simulink model "AN_Simulink_Model_v1_fil"  (R2019b)
settings: Solver=VariableStepAuto  StartTime=0.0  StopTime=testtime  RelTol=1e-3
InitFcn:
  | AN_InitFcn_Callback
StopFcn:
  | AN_StopFcn_Callback
undefined symbols (not defined in the file or in its folder): tdres
libraries: hdlmdlgenlib x193, simulink x4, fillib x1, dspsrcs4 x1
(part 4 of 6)

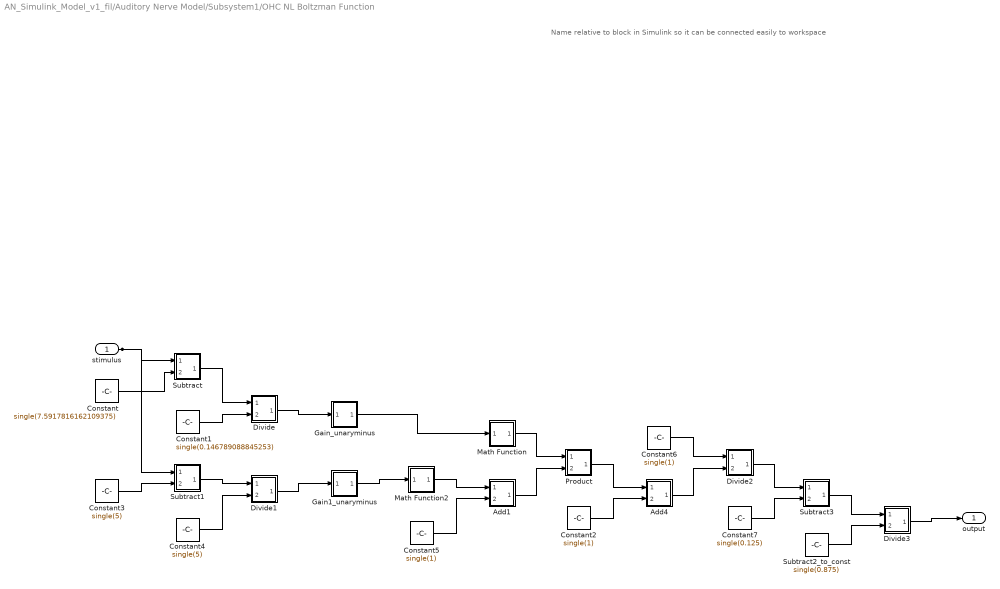
== system AN_Simulink_Model_v1_fil/Auditory Nerve Model/Subsystem1/OHC NL Boltzman Function ==
  note: Name relative to block in Simulink so it can be connected easily to workspace
  stimulus : Inport  OutDataTypeStr=single  PortDimensions=1  SampleTime=2.08333333333333e-05
  Add1 : Subsystem
      mask Display: disp('NFP\nadd');
  Add4 : Subsystem
      mask Display: disp('NFP\nadd');
  Constant : Constant  Value=single(7.5917816162109375)  OutDataTypeStr=single  SampleTime=-1
  Constant1 : Constant  Value=single(0.146789088845253)  OutDataTypeStr=single  SampleTime=-1
  Constant2 : Constant  Value=single(1)  OutDataTypeStr=single  SampleTime=-1
  Constant3 : Constant  Value=single(5)  OutDataTypeStr=single  SampleTime=-1
  Constant4 : Constant  Value=single(5)  OutDataTypeStr=single  SampleTime=-1
  Constant5 : Constant  Value=single(1)  OutDataTypeStr=single  SampleTime=-1
  Constant6 : Constant  Value=single(1)  OutDataTypeStr=single  SampleTime=-1
  Constant7 : Constant  Value=single(0.125)  OutDataTypeStr=single  SampleTime=-1
  Divide : Subsystem
      mask Display: disp('NFP\nmul');
  Divide1 : Subsystem
      mask Display: disp('NFP\nmul');
  Divide2 : Subsystem
      mask Display: disp('NFP\nmul');
  Divide3 : Subsystem
      mask Display: disp('NFP\nmul');
  Gain1_unaryminus : Subsystem
      mask Display: disp('NFP\numinus');
  Gain_unaryminus : Subsystem
      mask Display: disp('NFP\numinus');
  Math Function : Subsystem
      mask Display: disp('NFP\nmath');
  Math Function2 : Subsystem
      mask Display: disp('NFP\nmath');
  Product : Subsystem
      mask Display: disp('NFP\nmul');
  Subtract : Subsystem
      mask Display: disp('NFP\nadd');
  Subtract1 : Subsystem
      mask Display: disp('NFP\nadd');
  Subtract2_to_const : Constant  Value=single(0.875)  OutDataTypeStr=single  SampleTime=-1
  Subtract3 : Subsystem
      mask Display: disp('NFP\nadd');
  output : Outport  VectorParamsAs1DForOutWhenUnconnected=off
  wires:
  Subtract3/1(Out1) -> Divide3/1(In1)
  Subtract1/1(Out1) -> Divide1/1(In1)
  Subtract/1(Out1) -> Divide/1(In1)
  Product/1(Out1) -> Add4/1(In1)
  Math Function2/1(Out1) -> Add1/1(In1)
  Math Function/1(Out1) -> Product/1(In1)
  Divide3/1(Out1) -> output/1
  Divide2/1(Out1) -> Subtract3/1(In1)
  Divide1/1(Out1) -> Gain1_unaryminus/1(In1)
  Divide/1(Out1) -> Gain_unaryminus/1(In1)
  Add4/1(Out1) -> Divide2/2(In2)
  Add1/1(Out1) -> Product/2(In2)
  Gain1_unaryminus/1(Out1) -> Math Function2/1(In1)
  Gain_unaryminus/1(Out1) -> Math Function/1(In1)
  Subtract2_to_const/1 -> Divide3/2(In2)
  Constant7/1 -> Subtract3/2(In2)
  Constant6/1 -> Divide2/1(In1)
  Constant5/1 -> Add1/2(In2)
  Constant4/1 -> Divide1/2(In2)
  Constant3/1 -> Subtract1/2(In2)
  Constant2/1 -> Add4/2(In2)
  Constant1/1 -> Divide/2(In2)
  Constant/1 -> Subtract/2(In2)
  stimulus/1 -> Subtract/1(In1), Subtract1/1(In1)

== system AN_Simulink_Model_v1_fil/Compare/Assert_ihcout/RelErrCheck ==
  In1 : Inport
  In2 : Inport  Port=2
  "RelativeErrorCheck " : MATLAB Function  TreatAsAtomicUnit=on
  Out1 : Outport  VectorParamsAs1DForOutWhenUnconnected=off
  wires:
  In2/1 -> "RelativeErrorCheck "/2(R)
  In1/1 -> "RelativeErrorCheck "/1(P)
  "RelativeErrorCheck "/1(y) -> Out1/1

== system AN_Simulink_Model_v1_fil/Auditory Nerve Model/C1 Chirp Filter/C1 FIlter/Gain10_unaryminus ==
  In1 : Inport
  Gain10_unaryminus : UnaryMinus  SampleTime=2.08333333333333e-05
  Out1 : Outport
  wires:
  Gain10_unaryminus/1 -> Out1/1
  In1/1 -> Gain10_unaryminus/1

== system AN_Simulink_Model_v1_fil/Auditory Nerve Model/C1 Chirp Filter/C1 FIlter/Gain11_unaryminus ==
  In1 : Inport
  Gain11_unaryminus : UnaryMinus  SampleTime=2.08333333333333e-05
  Out1 : Outport
  wires:
  Gain11_unaryminus/1 -> Out1/1
  In1/1 -> Gain11_unaryminus/1

== system AN_Simulink_Model_v1_fil/Auditory Nerve Model/C1 Chirp Filter/C1 FIlter/Gain1_unaryminus ==
  In1 : Inport
  Gain1_unaryminus : UnaryMinus  SampleTime=2.08333333333333e-05
  Out1 : Outport
  wires:
  Gain1_unaryminus/1 -> Out1/1
  In1/1 -> Gain1_unaryminus/1

== system AN_Simulink_Model_v1_fil/Auditory Nerve Model/C1 Chirp Filter/C1 FIlter/Gain2_unaryminus ==
  In1 : Inport
  Gain2_unaryminus : UnaryMinus  SampleTime=2.08333333333333e-05
  Out1 : Outport
  wires:
  Gain2_unaryminus/1 -> Out1/1
  In1/1 -> Gain2_unaryminus/1

== system AN_Simulink_Model_v1_fil/Auditory Nerve Model/C1 Chirp Filter/C1 FIlter/Gain3_unaryminus ==
  In1 : Inport
  Gain3_unaryminus : UnaryMinus  SampleTime=2.08333333333333e-05
  Out1 : Outport
  wires:
  Gain3_unaryminus/1 -> Out1/1
  In1/1 -> Gain3_unaryminus/1

== system AN_Simulink_Model_v1_fil/Auditory Nerve Model/C1 Chirp Filter/C1 FIlter/Gain4_unaryminus ==
  In1 : Inport
  Gain4_unaryminus : UnaryMinus  SampleTime=2.08333333333333e-05
  Out1 : Outport
  wires:
  Gain4_unaryminus/1 -> Out1/1
  In1/1 -> Gain4_unaryminus/1

== system AN_Simulink_Model_v1_fil/Auditory Nerve Model/C1 Chirp Filter/C1 FIlter/Gain5_unaryminus ==
  In1 : Inport
  Gain5_unaryminus : UnaryMinus  SampleTime=2.08333333333333e-05
  Out1 : Outport
  wires:
  Gain5_unaryminus/1 -> Out1/1
  In1/1 -> Gain5_unaryminus/1

== system AN_Simulink_Model_v1_fil/Auditory Nerve Model/C1 Chirp Filter/C1 FIlter/Gain7_unaryminus ==
  In1 : Inport
  Gain7_unaryminus : UnaryMinus  SampleTime=2.08333333333333e-05
  Out1 : Outport
  wires:
  Gain7_unaryminus/1 -> Out1/1
  In1/1 -> Gain7_unaryminus/1

== system AN_Simulink_Model_v1_fil/Auditory Nerve Model/C1 Chirp Filter/C1 FIlter/Gain8_unaryminus ==
  In1 : Inport
  Gain8_unaryminus : UnaryMinus  SampleTime=2.08333333333333e-05
  Out1 : Outport
  wires:
  Gain8_unaryminus/1 -> Out1/1
  In1/1 -> Gain8_unaryminus/1

== system AN_Simulink_Model_v1_fil/Auditory Nerve Model/C1 Chirp Filter/C1 FIlter/Gain9_unaryminus ==
  In1 : Inport
  Gain9_unaryminus : UnaryMinus  SampleTime=2.08333333333333e-05
  Out1 : Outport
  wires:
  Gain9_unaryminus/1 -> Out1/1
  In1/1 -> Gain9_unaryminus/1

== system AN_Simulink_Model_v1_fil/Auditory Nerve Model/C1 Chirp Filter/C1 FIlter/Product ==
  In1 : Inport
  In2 : Inport  Port=2
  Product : Product  Inputs=**  OutDataTypeStr=single  SampleTime=2.08333333333333e-05
  Out1 : Outport
  wires:
  Product/1 -> Out1/1
  In2/1 -> Product/2
  In1/1 -> Product/1

== system AN_Simulink_Model_v1_fil/Auditory Nerve Model/C1 Chirp Filter/C1 FIlter/Product1 ==
  In1 : Inport
  In2 : Inport  Port=2
  Product1 : Product  Inputs=**  OutDataTypeStr=single  SampleTime=2.08333333333333e-05
  Out1 : Outport
  wires:
  Product1/1 -> Out1/1
  In2/1 -> Product1/2
  In1/1 -> Product1/1

== system AN_Simulink_Model_v1_fil/Auditory Nerve Model/C1 Chirp Filter/C1 FIlter/Product10 ==
  In1 : Inport
  In2 : Inport  Port=2
  Product10 : Product  Inputs=**  OutDataTypeStr=single  SampleTime=2.08333333333333e-05
  Out1 : Outport
  wires:
  Product10/1 -> Out1/1
  In2/1 -> Product10/2
  In1/1 -> Product10/1

== system AN_Simulink_Model_v1_fil/Auditory Nerve Model/C1 Chirp Filter/C1 FIlter/Product11 ==
  In1 : Inport
  In2 : Inport  Port=2
  Product11 : Product  Inputs=**  OutDataTypeStr=single  SampleTime=2.08333333333333e-05
  Out1 : Outport
  wires:
  Product11/1 -> Out1/1
  In2/1 -> Product11/2
  In1/1 -> Product11/1

== system AN_Simulink_Model_v1_fil/Auditory Nerve Model/C1 Chirp Filter/C1 FIlter/Product12 ==
  In1 : Inport
  In2 : Inport  Port=2
  Product12 : Product  Inputs=**  OutDataTypeStr=single  SampleTime=2.08333333333333e-05
  Out1 : Outport
  wires:
  Product12/1 -> Out1/1
  In2/1 -> Product12/2
  In1/1 -> Product12/1

== system AN_Simulink_Model_v1_fil/Auditory Nerve Model/C1 Chirp Filter/C1 FIlter/Product13 ==
  In1 : Inport
  In2 : Inport  Port=2
  Product13 : Product  Inputs=**  OutDataTypeStr=single  SampleTime=2.08333333333333e-05
  Out1 : Outport
  wires:
  Product13/1 -> Out1/1
  In2/1 -> Product13/2
  In1/1 -> Product13/1

== system AN_Simulink_Model_v1_fil/Auditory Nerve Model/C1 Chirp Filter/C1 FIlter/Product14 ==
  In1 : Inport
  In2 : Inport  Port=2
  Product14 : Product  Inputs=**  OutDataTypeStr=single  SampleTime=2.08333333333333e-05
  Out1 : Outport
  wires:
  Product14/1 -> Out1/1
  In2/1 -> Product14/2
  In1/1 -> Product14/1

== system AN_Simulink_Model_v1_fil/Auditory Nerve Model/C1 Chirp Filter/C1 FIlter/Product15 ==
  In1 : Inport
  In2 : Inport  Port=2
  Product15 : Product  Inputs=**  OutDataTypeStr=single  SampleTime=2.08333333333333e-05
  Out1 : Outport
  wires:
  Product15/1 -> Out1/1
  In2/1 -> Product15/2
  In1/1 -> Product15/1

== system AN_Simulink_Model_v1_fil/Auditory Nerve Model/C1 Chirp Filter/C1 FIlter/Product16 ==
  In1 : Inport
  In2 : Inport  Port=2
  Product16 : Product  Inputs=**  OutDataTypeStr=single  SampleTime=2.08333333333333e-05
  Out1 : Outport
  wires:
  Product16/1 -> Out1/1
  In2/1 -> Product16/2
  In1/1 -> Product16/1

== system AN_Simulink_Model_v1_fil/Auditory Nerve Model/C1 Chirp Filter/C1 FIlter/Product17 ==
  In1 : Inport
  In2 : Inport  Port=2
  Product17 : Product  Inputs=**  OutDataTypeStr=single  SampleTime=2.08333333333333e-05
  Out1 : Outport
  wires:
  Product17/1 -> Out1/1
  In2/1 -> Product17/2
  In1/1 -> Product17/1

== system AN_Simulink_Model_v1_fil/Auditory Nerve Model/C1 Chirp Filter/C1 FIlter/Product18 ==
  In1 : Inport
  In2 : Inport  Port=2
  Product18 : Product  Inputs=**  OutDataTypeStr=single  SampleTime=2.08333333333333e-05
  Out1 : Outport
  wires:
  Product18/1 -> Out1/1
  In2/1 -> Product18/2
  In1/1 -> Product18/1

== system AN_Simulink_Model_v1_fil/Auditory Nerve Model/C1 Chirp Filter/C1 FIlter/Product19 ==
  In1 : Inport
  In2 : Inport  Port=2
  Product19 : Product  Inputs=**  OutDataTypeStr=single  SampleTime=2.08333333333333e-05
  Out1 : Outport
  wires:
  Product19/1 -> Out1/1
  In2/1 -> Product19/2
  In1/1 -> Product19/1

== system AN_Simulink_Model_v1_fil/Auditory Nerve Model/C1 Chirp Filter/C1 FIlter/Product2 ==
  In1 : Inport
  In2 : Inport  Port=2
  Product2 : Product  Inputs=**  OutDataTypeStr=single  SampleTime=2.08333333333333e-05
  Out1 : Outport
  wires:
  Product2/1 -> Out1/1
  In2/1 -> Product2/2
  In1/1 -> Product2/1

== system AN_Simulink_Model_v1_fil/Auditory Nerve Model/C1 Chirp Filter/C1 FIlter/Product20 ==
  In1 : Inport
  In2 : Inport  Port=2
  Product20 : Product  Inputs=**  OutDataTypeStr=single  SampleTime=2.08333333333333e-05
  Out1 : Outport
  wires:
  Product20/1 -> Out1/1
  In2/1 -> Product20/2
  In1/1 -> Product20/1

== system AN_Simulink_Model_v1_fil/Auditory Nerve Model/C1 Chirp Filter/C1 FIlter/Product21 ==
  In1 : Inport
  In2 : Inport  Port=2
  Product21 : Product  Inputs=**  OutDataTypeStr=single  SampleTime=2.08333333333333e-05
  Out1 : Outport
  wires:
  Product21/1 -> Out1/1
  In2/1 -> Product21/2
  In1/1 -> Product21/1

== system AN_Simulink_Model_v1_fil/Auditory Nerve Model/C1 Chirp Filter/C1 FIlter/Product22 ==
  In1 : Inport
  In2 : Inport  Port=2
  Product22 : Product  Inputs=**  OutDataTypeStr=single  SampleTime=2.08333333333333e-05
  Out1 : Outport
  wires:
  Product22/1 -> Out1/1
  In2/1 -> Product22/2
  In1/1 -> Product22/1

== system AN_Simulink_Model_v1_fil/Auditory Nerve Model/C1 Chirp Filter/C1 FIlter/Product23 ==
  In1 : Inport
  In2 : Inport  Port=2
  Product23 : Product  Inputs=**  OutDataTypeStr=single  SampleTime=2.08333333333333e-05
  Out1 : Outport
  wires:
  Product23/1 -> Out1/1
  In2/1 -> Product23/2
  In1/1 -> Product23/1

== system AN_Simulink_Model_v1_fil/Auditory Nerve Model/C1 Chirp Filter/C1 FIlter/Product24 ==
  In1 : Inport
  In2 : Inport  Port=2
  Product24 : Product  Inputs=**  OutDataTypeStr=single  SampleTime=2.08333333333333e-05
  Out1 : Outport
  wires:
  Product24/1 -> Out1/1
  In2/1 -> Product24/2
  In1/1 -> Product24/1

== system AN_Simulink_Model_v1_fil/Auditory Nerve Model/C1 Chirp Filter/C1 FIlter/Product25_to_gain ==
  In1 : Inport
  Product25_to_gain : Gain  Gain=single(0.25)
  Out1 : Outport
  wires:
  Product25_to_gain/1 -> Out1/1
  In1/1 -> Product25_to_gain/1

== system AN_Simulink_Model_v1_fil/Auditory Nerve Model/C1 Chirp Filter/C1 FIlter/Product26 ==
  In1 : Inport
  In2 : Inport  Port=2
  Product26 : Product  Inputs=**  OutDataTypeStr=single  SampleTime=2.08333333333333e-05
  Out1 : Outport
  wires:
  Product26/1 -> Out1/1
  In2/1 -> Product26/2
  In1/1 -> Product26/1

== system AN_Simulink_Model_v1_fil/Auditory Nerve Model/C1 Chirp Filter/C1 FIlter/Product3 ==
  In1 : Inport
  In2 : Inport  Port=2
  Product3 : Product  Inputs=**  OutDataTypeStr=single  SampleTime=2.08333333333333e-05
  Out1 : Outport
  wires:
  Product3/1 -> Out1/1
  In2/1 -> Product3/2
  In1/1 -> Product3/1

== system AN_Simulink_Model_v1_fil/Auditory Nerve Model/C1 Chirp Filter/C1 FIlter/Product4 ==
  In1 : Inport
  In2 : Inport  Port=2
  Product4 : Product  Inputs=**  OutDataTypeStr=single  SampleTime=2.08333333333333e-05
  Out1 : Outport
  wires:
  Product4/1 -> Out1/1
  In2/1 -> Product4/2
  In1/1 -> Product4/1

== system AN_Simulink_Model_v1_fil/Auditory Nerve Model/C1 Chirp Filter/C1 FIlter/Product5 ==
  In1 : Inport
  In2 : Inport  Port=2
  Product5 : Product  Inputs=**  OutDataTypeStr=single  SampleTime=2.08333333333333e-05
  Out1 : Outport
  wires:
  Product5/1 -> Out1/1
  In2/1 -> Product5/2
  In1/1 -> Product5/1

== system AN_Simulink_Model_v1_fil/Auditory Nerve Model/C1 Chirp Filter/C1 FIlter/Product6 ==
  In1 : Inport
  In2 : Inport  Port=2
  Product6 : Product  Inputs=**  OutDataTypeStr=single  SampleTime=2.08333333333333e-05
  Out1 : Outport
  wires:
  Product6/1 -> Out1/1
  In2/1 -> Product6/2
  In1/1 -> Product6/1

== system AN_Simulink_Model_v1_fil/Auditory Nerve Model/C1 Chirp Filter/C1 FIlter/Product7 ==
  In1 : Inport
  In2 : Inport  Port=2
  Product7 : Product  Inputs=**  OutDataTypeStr=single  SampleTime=2.08333333333333e-05
  Out1 : Outport
  wires:
  Product7/1 -> Out1/1
  In2/1 -> Product7/2
  In1/1 -> Product7/1

== system AN_Simulink_Model_v1_fil/Auditory Nerve Model/C1 Chirp Filter/C1 FIlter/Product8 ==
  In1 : Inport
  In2 : Inport  Port=2
  Product8 : Product  Inputs=**  OutDataTypeStr=single  SampleTime=2.08333333333333e-05
  Out1 : Outport
  wires:
  Product8/1 -> Out1/1
  In2/1 -> Product8/2
  In1/1 -> Product8/1

== system AN_Simulink_Model_v1_fil/Auditory Nerve Model/C1 Chirp Filter/C1 FIlter/Product9 ==
  In1 : Inport
  In2 : Inport  Port=2
  Product9 : Product  Inputs=**  OutDataTypeStr=single  SampleTime=2.08333333333333e-05
  Out1 : Outport
  wires:
  Product9/1 -> Out1/1
  In2/1 -> Product9/2
  In1/1 -> Product9/1

== system AN_Simulink_Model_v1_fil/Auditory Nerve Model/C1 Chirp Filter/C1 FIlter/Sum ==
  In1 : Inport
  In2 : Inport  Port=2
  Sum : Sum  OutDataTypeStr=single  SampleTime=2.08333333333333e-05  SaturateOnIntegerOverflow=on  InputSameDT=on
  Out1 : Outport
  wires:
  Sum/1 -> Out1/1
  In2/1 -> Sum/2
  In1/1 -> Sum/1

== system AN_Simulink_Model_v1_fil/Auditory Nerve Model/C1 Chirp Filter/C1 FIlter/Sum1 ==
  In1 : Inport
  In2 : Inport  Port=2
  Sum1 : Sum  OutDataTypeStr=single  SampleTime=2.08333333333333e-05  SaturateOnIntegerOverflow=on  InputSameDT=on
  Out1 : Outport
  wires:
  Sum1/1 -> Out1/1
  In2/1 -> Sum1/2
  In1/1 -> Sum1/1

== system AN_Simulink_Model_v1_fil/Auditory Nerve Model/C1 Chirp Filter/C1 FIlter/Sum10 ==
  In1 : Inport
  In2 : Inport  Port=2
  Sum10 : Sum  OutDataTypeStr=single  SampleTime=2.08333333333333e-05  SaturateOnIntegerOverflow=on  InputSameDT=on
  Out1 : Outport
  wires:
  Sum10/1 -> Out1/1
  In2/1 -> Sum10/2
  In1/1 -> Sum10/1

== system AN_Simulink_Model_v1_fil/Auditory Nerve Model/C1 Chirp Filter/C1 FIlter/Sum11 ==
  In1 : Inport
  In2 : Inport  Port=2
  Sum11 : Sum  OutDataTypeStr=single  SampleTime=2.08333333333333e-05  SaturateOnIntegerOverflow=on  InputSameDT=on
  Out1 : Outport
  wires:
  Sum11/1 -> Out1/1
  In2/1 -> Sum11/2
  In1/1 -> Sum11/1

== system AN_Simulink_Model_v1_fil/Auditory Nerve Model/C1 Chirp Filter/C1 FIlter/Sum12 ==
  In1 : Inport
  In2 : Inport  Port=2
  Sum12 : Sum  OutDataTypeStr=single  SampleTime=2.08333333333333e-05  SaturateOnIntegerOverflow=on  InputSameDT=on
  Out1 : Outport
  wires:
  Sum12/1 -> Out1/1
  In2/1 -> Sum12/2
  In1/1 -> Sum12/1

== system AN_Simulink_Model_v1_fil/Auditory Nerve Model/C1 Chirp Filter/C1 FIlter/Sum13 ==
  In1 : Inport
  In2 : Inport  Port=2
  Sum13 : Sum  OutDataTypeStr=single  SampleTime=2.08333333333333e-05  SaturateOnIntegerOverflow=on  InputSameDT=on
  Out1 : Outport
  wires:
  Sum13/1 -> Out1/1
  In2/1 -> Sum13/2
  In1/1 -> Sum13/1

== system AN_Simulink_Model_v1_fil/Auditory Nerve Model/C1 Chirp Filter/C1 FIlter/Sum14 ==
  In1 : Inport
  In2 : Inport  Port=2
  Sum14 : Sum  OutDataTypeStr=single  SampleTime=2.08333333333333e-05  SaturateOnIntegerOverflow=on  InputSameDT=on
  Out1 : Outport
  wires:
  Sum14/1 -> Out1/1
  In2/1 -> Sum14/2
  In1/1 -> Sum14/1

== system AN_Simulink_Model_v1_fil/Auditory Nerve Model/C1 Chirp Filter/C1 FIlter/Sum15 ==
  In1 : Inport
  In2 : Inport  Port=2
  Sum15 : Sum  OutDataTypeStr=single  SampleTime=2.08333333333333e-05  SaturateOnIntegerOverflow=on  InputSameDT=on
  Out1 : Outport
  wires:
  Sum15/1 -> Out1/1
  In2/1 -> Sum15/2
  In1/1 -> Sum15/1

== system AN_Simulink_Model_v1_fil/Auditory Nerve Model/C1 Chirp Filter/C1 FIlter/Sum16 ==
  In1 : Inport
  In2 : Inport  Port=2
  Sum16 : Sum  OutDataTypeStr=single  SampleTime=2.08333333333333e-05  SaturateOnIntegerOverflow=on  InputSameDT=on
  Out1 : Outport
  wires:
  Sum16/1 -> Out1/1
  In2/1 -> Sum16/2
  In1/1 -> Sum16/1

== system AN_Simulink_Model_v1_fil/Auditory Nerve Model/C1 Chirp Filter/C1 FIlter/Sum17 ==
  In1 : Inport
  In2 : Inport  Port=2
  Sum17 : Sum  OutDataTypeStr=single  SampleTime=2.08333333333333e-05  SaturateOnIntegerOverflow=on  InputSameDT=on
  Out1 : Outport
  wires:
  Sum17/1 -> Out1/1
  In2/1 -> Sum17/2
  In1/1 -> Sum17/1

== system AN_Simulink_Model_v1_fil/Auditory Nerve Model/C1 Chirp Filter/C1 FIlter/Sum18 ==
  In1 : Inport
  In2 : Inport  Port=2
  Sum18 : Sum  OutDataTypeStr=single  SampleTime=2.08333333333333e-05  SaturateOnIntegerOverflow=on  InputSameDT=on
  Out1 : Outport
  wires:
  Sum18/1 -> Out1/1
  In2/1 -> Sum18/2
  In1/1 -> Sum18/1

== system AN_Simulink_Model_v1_fil/Auditory Nerve Model/C1 Chirp Filter/C1 FIlter/Sum19 ==
  In1 : Inport
  In2 : Inport  Port=2
  Sum19 : Sum  OutDataTypeStr=single  SampleTime=2.08333333333333e-05  SaturateOnIntegerOverflow=on  InputSameDT=on
  Out1 : Outport
  wires:
  Sum19/1 -> Out1/1
  In2/1 -> Sum19/2
  In1/1 -> Sum19/1

== system AN_Simulink_Model_v1_fil/Auditory Nerve Model/C1 Chirp Filter/C1 FIlter/Sum2 ==
  In1 : Inport
  In2 : Inport  Port=2
  Sum2 : Sum  OutDataTypeStr=single  SampleTime=2.08333333333333e-05  SaturateOnIntegerOverflow=on  InputSameDT=on
  Out1 : Outport
  wires:
  Sum2/1 -> Out1/1
  In2/1 -> Sum2/2
  In1/1 -> Sum2/1

== system AN_Simulink_Model_v1_fil/Auditory Nerve Model/C1 Chirp Filter/C1 FIlter/Sum3 ==
  In1 : Inport
  In2 : Inport  Port=2
  Sum3 : Sum  OutDataTypeStr=single  SampleTime=2.08333333333333e-05  SaturateOnIntegerOverflow=on  InputSameDT=on
  Out1 : Outport
  wires:
  Sum3/1 -> Out1/1
  In2/1 -> Sum3/2
  In1/1 -> Sum3/1

== system AN_Simulink_Model_v1_fil/Auditory Nerve Model/C1 Chirp Filter/C1 FIlter/Sum4 ==
  In1 : Inport
  In2 : Inport  Port=2
  Sum4 : Sum  OutDataTypeStr=single  SampleTime=2.08333333333333e-05  SaturateOnIntegerOverflow=on  InputSameDT=on
  Out1 : Outport
  wires:
  Sum4/1 -> Out1/1
  In2/1 -> Sum4/2
  In1/1 -> Sum4/1

== system AN_Simulink_Model_v1_fil/Auditory Nerve Model/C1 Chirp Filter/C1 FIlter/Sum5 ==
  In1 : Inport
  In2 : Inport  Port=2
  Sum5 : Sum  OutDataTypeStr=single  SampleTime=2.08333333333333e-05  SaturateOnIntegerOverflow=on  InputSameDT=on
  Out1 : Outport
  wires:
  Sum5/1 -> Out1/1
  In2/1 -> Sum5/2
  In1/1 -> Sum5/1

== system AN_Simulink_Model_v1_fil/Auditory Nerve Model/C1 Chirp Filter/C1 FIlter/Sum6 ==
  In1 : Inport
  In2 : Inport  Port=2
  Sum6 : Sum  OutDataTypeStr=single  SampleTime=2.08333333333333e-05  SaturateOnIntegerOverflow=on  InputSameDT=on
  Out1 : Outport
  wires:
  Sum6/1 -> Out1/1
  In2/1 -> Sum6/2
  In1/1 -> Sum6/1

== system AN_Simulink_Model_v1_fil/Auditory Nerve Model/C1 Chirp Filter/C1 FIlter/Sum7 ==
  In1 : Inport
  In2 : Inport  Port=2
  Sum7 : Sum  OutDataTypeStr=single  SampleTime=2.08333333333333e-05  SaturateOnIntegerOverflow=on  InputSameDT=on
  Out1 : Outport
  wires:
  Sum7/1 -> Out1/1
  In2/1 -> Sum7/2
  In1/1 -> Sum7/1

== system AN_Simulink_Model_v1_fil/Auditory Nerve Model/C1 Chirp Filter/C1 FIlter/Sum8 ==
  In1 : Inport
  In2 : Inport  Port=2
  Sum8 : Sum  OutDataTypeStr=single  SampleTime=2.08333333333333e-05  SaturateOnIntegerOverflow=on  InputSameDT=on
  Out1 : Outport
  wires:
  Sum8/1 -> Out1/1
  In2/1 -> Sum8/2
  In1/1 -> Sum8/1

== system AN_Simulink_Model_v1_fil/Auditory Nerve Model/C1 Chirp Filter/C1 FIlter/Sum9 ==
  In1 : Inport
  In2 : Inport  Port=2
  Sum9 : Sum  OutDataTypeStr=single  SampleTime=2.08333333333333e-05  SaturateOnIntegerOverflow=on  InputSameDT=on
  Out1 : Outport
  wires:
  Sum9/1 -> Out1/1
  In2/1 -> Sum9/2
  In1/1 -> Sum9/1

== system AN_Simulink_Model_v1_fil/Auditory Nerve Model/C1 Chirp Filter/Calculate rsigma/Reciprocal1_recip ==
  In1 : Inport
  Reciprocal1_recip : Math  Operator=reciprocal  SampleTime=2.08333333333333e-05  SaturateOnIntegerOverflow=on
  Out1 : Outport
  wires:
  Reciprocal1_recip/1 -> Out1/1
  In1/1 -> Reciprocal1_recip/1

== system AN_Simulink_Model_v1_fil/Auditory Nerve Model/C1 Chirp Filter/Calculate rsigma/Reciprocal_recip ==
  In1 : Inport
  Reciprocal_recip : Math  Operator=reciprocal  SampleTime=2.08333333333333e-05  SaturateOnIntegerOverflow=on
  Out1 : Outport
  wires:
  Reciprocal_recip/1 -> Out1/1
  In1/1 -> Reciprocal_recip/1

== system AN_Simulink_Model_v1_fil/Auditory Nerve Model/C1 Chirp Filter/Calculate rsigma/Subtract ==
  In1 : Inport
  In2 : Inport  Port=2
  Subtract : Sum  Inputs=+-  OutDataTypeStr=single  SampleTime=2.08333333333333e-05  SaturateOnIntegerOverflow=on  InputSameDT=on
  Out1 : Outport
  wires:
  Subtract/1 -> Out1/1
  In2/1 -> Subtract/2
  In1/1 -> Subtract/1

== system AN_Simulink_Model_v1_fil/Auditory Nerve Model/C1 Chirp Filter/Get C1 Coefficients/Add10 ==
  In1 : Inport
  In2 : Inport  Port=2
  Add10 : Sum  OutDataTypeStr=single  SampleTime=2.08333333333333e-05  SaturateOnIntegerOverflow=on  InputSameDT=on
  Out1 : Outport
  wires:
  Add10/1 -> Out1/1
  In2/1 -> Add10/2
  In1/1 -> Add10/1

== system AN_Simulink_Model_v1_fil/Auditory Nerve Model/C1 Chirp Filter/Get C1 Coefficients/Add11 ==
  In1 : Inport
  In2 : Inport  Port=2
  Add11 : Sum  OutDataTypeStr=single  SampleTime=2.08333333333333e-05  SaturateOnIntegerOverflow=on  InputSameDT=on
  Out1 : Outport
  wires:
  Add11/1 -> Out1/1
  In2/1 -> Add11/2
  In1/1 -> Add11/1

== system AN_Simulink_Model_v1_fil/Auditory Nerve Model/C1 Chirp Filter/Get C1 Coefficients/Add12_stage2 ==
  In1 : Inport
  In2 : Inport  Port=2
  Add12_stage2 : Sum  Inputs=+-  OutDataTypeStr=single  SampleTime=2.08333333333333e-05  SaturateOnIntegerOverflow=on  InputSameDT=on
  Out1 : Outport
  wires:
  Add12_stage2/1 -> Out1/1
  In2/1 -> Add12_stage2/2
  In1/1 -> Add12_stage2/1

== system AN_Simulink_Model_v1_fil/Auditory Nerve Model/C1 Chirp Filter/Get C1 Coefficients/Add12_stage3 ==
  In1 : Inport
  In2 : Inport  Port=2
  Add12_stage3 : Sum  Inputs=+-  OutDataTypeStr=single  SampleTime=2.08333333333333e-05  SaturateOnIntegerOverflow=on  InputSameDT=on
  Out1 : Outport
  wires:
  Add12_stage3/1 -> Out1/1
  In2/1 -> Add12_stage3/2
  In1/1 -> Add12_stage3/1

== system AN_Simulink_Model_v1_fil/Auditory Nerve Model/C1 Chirp Filter/Get C1 Coefficients/Add13_stage2 ==
  In1 : Inport
  In2 : Inport  Port=2
  Add13_stage2 : Sum  Inputs=+-  OutDataTypeStr=single  SampleTime=2.08333333333333e-05  SaturateOnIntegerOverflow=on  InputSameDT=on
  Out1 : Outport
  wires:
  Add13_stage2/1 -> Out1/1
  In2/1 -> Add13_stage2/2
  In1/1 -> Add13_stage2/1

== system AN_Simulink_Model_v1_fil/Auditory Nerve Model/C1 Chirp Filter/Get C1 Coefficients/Add13_stage3 ==
  In1 : Inport
  In2 : Inport  Port=2
  Add13_stage3 : Sum  Inputs=+-  OutDataTypeStr=single  SampleTime=2.08333333333333e-05  SaturateOnIntegerOverflow=on  InputSameDT=on
  Out1 : Outport
  wires:
  Add13_stage3/1 -> Out1/1
  In2/1 -> Add13_stage3/2
  In1/1 -> Add13_stage3/1

== system AN_Simulink_Model_v1_fil/Auditory Nerve Model/C1 Chirp Filter/Get C1 Coefficients/Add14_stage2 ==
  In1 : Inport
  In2 : Inport  Port=2
  Add14_stage2 : Sum  Inputs=+-  OutDataTypeStr=single  SampleTime=2.08333333333333e-05  SaturateOnIntegerOverflow=on  InputSameDT=on
  Out1 : Outport
  wires:
  Add14_stage2/1 -> Out1/1
  In2/1 -> Add14_stage2/2
  In1/1 -> Add14_stage2/1

== system AN_Simulink_Model_v1_fil/Auditory Nerve Model/C1 Chirp Filter/Get C1 Coefficients/Add14_stage3 ==
  In1 : Inport
  In2 : Inport  Port=2
  Add14_stage3 : Sum  Inputs=+-  OutDataTypeStr=single  SampleTime=2.08333333333333e-05  SaturateOnIntegerOverflow=on  InputSameDT=on
  Out1 : Outport
  wires:
  Add14_stage3/1 -> Out1/1
  In2/1 -> Add14_stage3/2
  In1/1 -> Add14_stage3/1

== system AN_Simulink_Model_v1_fil/Auditory Nerve Model/C1 Chirp Filter/Get C1 Coefficients/Add15 ==
  In1 : Inport
  In2 : Inport  Port=2
  Add15 : Sum  OutDataTypeStr=single  SampleTime=2.08333333333333e-05  SaturateOnIntegerOverflow=on  InputSameDT=on
  Out1 : Outport
  wires:
  Add15/1 -> Out1/1
  In2/1 -> Add15/2
  In1/1 -> Add15/1

== system AN_Simulink_Model_v1_fil/Auditory Nerve Model/C1 Chirp Filter/Get C1 Coefficients/Add16 ==
  In1 : Inport
  In2 : Inport  Port=2
  Add16 : Sum  OutDataTypeStr=single  SampleTime=2.08333333333333e-05  SaturateOnIntegerOverflow=on  InputSameDT=on
  Out1 : Outport
  wires:
  Add16/1 -> Out1/1
  In2/1 -> Add16/2
  In1/1 -> Add16/1

== system AN_Simulink_Model_v1_fil/Auditory Nerve Model/C1 Chirp Filter/Get C1 Coefficients/Add17 ==
  In1 : Inport
  In2 : Inport  Port=2
  Add17 : Sum  OutDataTypeStr=single  SampleTime=2.08333333333333e-05  SaturateOnIntegerOverflow=on  InputSameDT=on
  Out1 : Outport
  wires:
  Add17/1 -> Out1/1
  In2/1 -> Add17/2
  In1/1 -> Add17/1

== system AN_Simulink_Model_v1_fil/Auditory Nerve Model/C1 Chirp Filter/Get C1 Coefficients/Add4_stage2 ==
  In1 : Inport
  In2 : Inport  Port=2
  Add4_stage2 : Sum  OutDataTypeStr=single  SampleTime=2.08333333333333e-05  SaturateOnIntegerOverflow=on  InputSameDT=on
  Out1 : Outport
  wires:
  Add4_stage2/1 -> Out1/1
  In2/1 -> Add4_stage2/2
  In1/1 -> Add4_stage2/1

== system AN_Simulink_Model_v1_fil/Auditory Nerve Model/C1 Chirp Filter/Get C1 Coefficients/Add4_stage3 ==
  In1 : Inport
  In2 : Inport  Port=2
  Add4_stage3 : Sum  OutDataTypeStr=single  SampleTime=2.08333333333333e-05  SaturateOnIntegerOverflow=on  InputSameDT=on
  Out1 : Outport
  wires:
  Add4_stage3/1 -> Out1/1
  In2/1 -> Add4_stage3/2
  In1/1 -> Add4_stage3/1

== system AN_Simulink_Model_v1_fil/Auditory Nerve Model/C1 Chirp Filter/Get C1 Coefficients/Add5 ==
  In1 : Inport
  In2 : Inport  Port=2
  Add5 : Sum  Inputs=--  OutDataTypeStr=single  SampleTime=2.08333333333333e-05  SaturateOnIntegerOverflow=on  InputSameDT=on
  Out1 : Outport
  wires:
  Add5/1 -> Out1/1
  In2/1 -> Add5/2
  In1/1 -> Add5/1

== system AN_Simulink_Model_v1_fil/Auditory Nerve Model/C1 Chirp Filter/Get C1 Coefficients/Add6 ==
  In1 : Inport
  In2 : Inport  Port=2
  Add6 : Sum  OutDataTypeStr=single  SampleTime=2.08333333333333e-05  SaturateOnIntegerOverflow=on  InputSameDT=on
  Out1 : Outport
  wires:
  Add6/1 -> Out1/1
  In2/1 -> Add6/2
  In1/1 -> Add6/1

== system AN_Simulink_Model_v1_fil/Auditory Nerve Model/C1 Chirp Filter/Get C1 Coefficients/Add7 ==
  In1 : Inport
  In2 : Inport  Port=2
  Add7 : Sum  OutDataTypeStr=single  SampleTime=2.08333333333333e-05  SaturateOnIntegerOverflow=on  InputSameDT=on
  Out1 : Outport
  wires:
  Add7/1 -> Out1/1
  In2/1 -> Add7/2
  In1/1 -> Add7/1

== system AN_Simulink_Model_v1_fil/Auditory Nerve Model/C1 Chirp Filter/Get C1 Coefficients/Add8 ==
  In1 : Inport
  In2 : Inport  Port=2
  Add8 : Sum  OutDataTypeStr=single  SampleTime=2.08333333333333e-05  SaturateOnIntegerOverflow=on  InputSameDT=on
  Out1 : Outport
  wires:
  Add8/1 -> Out1/1
  In2/1 -> Add8/2
  In1/1 -> Add8/1

== system AN_Simulink_Model_v1_fil/Auditory Nerve Model/C1 Chirp Filter/Get C1 Coefficients/Add9 ==
  In1 : Inport
  In2 : Inport  Port=2
  Add9 : Sum  OutDataTypeStr=single  SampleTime=2.08333333333333e-05  SaturateOnIntegerOverflow=on  InputSameDT=on
  Out1 : Outport
  wires:
  Add9/1 -> Out1/1
  In2/1 -> Add9/2
  In1/1 -> Add9/1

== system AN_Simulink_Model_v1_fil/Auditory Nerve Model/C1 Chirp Filter/Get C1 Coefficients/Divide1 ==
  In1 : Inport
  In2 : Inport  Port=2
  Divide1 : Product  Inputs=*/  OutDataTypeStr=single  SampleTime=2.08333333333333e-05  SaturateOnIntegerOverflow=on  RndMeth=Zero
  Out1 : Outport
  wires:
  Divide1/1 -> Out1/1
  In2/1 -> Divide1/2
  In1/1 -> Divide1/1

== system AN_Simulink_Model_v1_fil/Auditory Nerve Model/C1 Chirp Filter/Get C1 Coefficients/Divide10 ==
  In1 : Inport
  In2 : Inport  Port=2
  Divide10 : Product  Inputs=*/  OutDataTypeStr=single  SampleTime=2.08333333333333e-05  SaturateOnIntegerOverflow=on  RndMeth=Zero
  Out1 : Outport
  wires:
  Divide10/1 -> Out1/1
  In2/1 -> Divide10/2
  In1/1 -> Divide10/1

== system AN_Simulink_Model_v1_fil/Auditory Nerve Model/C1 Chirp Filter/Get C1 Coefficients/Divide11 ==
  In1 : Inport
  In2 : Inport  Port=2
  Divide11 : Product  Inputs=*/  OutDataTypeStr=single  SampleTime=2.08333333333333e-05  SaturateOnIntegerOverflow=on  RndMeth=Zero
  Out1 : Outport
  wires:
  Divide11/1 -> Out1/1
  In2/1 -> Divide11/2
  In1/1 -> Divide11/1

== system AN_Simulink_Model_v1_fil/Auditory Nerve Model/C1 Chirp Filter/Get C1 Coefficients/Divide12 ==
  In1 : Inport
  In2 : Inport  Port=2
  Divide12 : Product  Inputs=*/  OutDataTypeStr=single  SampleTime=2.08333333333333e-05  SaturateOnIntegerOverflow=on  RndMeth=Zero
  Out1 : Outport
  wires:
  Divide12/1 -> Out1/1
  In2/1 -> Divide12/2
  In1/1 -> Divide12/1

== system AN_Simulink_Model_v1_fil/Auditory Nerve Model/C1 Chirp Filter/Get C1 Coefficients/Divide13 ==
  In1 : Inport
  In2 : Inport  Port=2
  Divide13 : Product  Inputs=*/  OutDataTypeStr=single  SampleTime=2.08333333333333e-05  SaturateOnIntegerOverflow=on  RndMeth=Zero
  Out1 : Outport
  wires:
  Divide13/1 -> Out1/1
  In2/1 -> Divide13/2
  In1/1 -> Divide13/1

== system AN_Simulink_Model_v1_fil/Auditory Nerve Model/C1 Chirp Filter/Get C1 Coefficients/Divide14 ==
  In1 : Inport
  In2 : Inport  Port=2
  Divide14 : Product  Inputs=*/  OutDataTypeStr=single  SampleTime=2.08333333333333e-05  SaturateOnIntegerOverflow=on  RndMeth=Zero
  Out1 : Outport
  wires:
  Divide14/1 -> Out1/1
  In2/1 -> Divide14/2
  In1/1 -> Divide14/1

== system AN_Simulink_Model_v1_fil/Auditory Nerve Model/C1 Chirp Filter/Get C1 Coefficients/Divide15 ==
  In1 : Inport
  In2 : Inport  Port=2
  Divide15 : Product  Inputs=*/  OutDataTypeStr=single  SampleTime=2.08333333333333e-05  SaturateOnIntegerOverflow=on  RndMeth=Zero
  Out1 : Outport
  wires:
  Divide15/1 -> Out1/1
  In2/1 -> Divide15/2
  In1/1 -> Divide15/1

== system AN_Simulink_Model_v1_fil/Auditory Nerve Model/C1 Chirp Filter/Get C1 Coefficients/Divide16 ==
  In1 : Inport
  In2 : Inport  Port=2
  Divide16 : Product  Inputs=*/  OutDataTypeStr=single  SampleTime=2.08333333333333e-05  SaturateOnIntegerOverflow=on  RndMeth=Zero
  Out1 : Outport
  wires:
  Divide16/1 -> Out1/1
  In2/1 -> Divide16/2
  In1/1 -> Divide16/1

== system AN_Simulink_Model_v1_fil/Auditory Nerve Model/C1 Chirp Filter/Get C1 Coefficients/Divide17 ==
  In1 : Inport
  In2 : Inport  Port=2
  Divide17 : Product  Inputs=*/  OutDataTypeStr=single  SampleTime=2.08333333333333e-05  SaturateOnIntegerOverflow=on  RndMeth=Zero
  Out1 : Outport
  wires:
  Divide17/1 -> Out1/1
  In2/1 -> Divide17/2
  In1/1 -> Divide17/1

== system AN_Simulink_Model_v1_fil/Auditory Nerve Model/C1 Chirp Filter/Get C1 Coefficients/Divide18 ==
  In1 : Inport
  In2 : Inport  Port=2
  Divide18 : Product  Inputs=*/  OutDataTypeStr=single  SampleTime=2.08333333333333e-05  SaturateOnIntegerOverflow=on  RndMeth=Zero
  Out1 : Outport
  wires:
  Divide18/1 -> Out1/1
  In2/1 -> Divide18/2
  In1/1 -> Divide18/1

== system AN_Simulink_Model_v1_fil/Auditory Nerve Model/C1 Chirp Filter/Get C1 Coefficients/Divide19 ==
  In1 : Inport
  In2 : Inport  Port=2
  Divide19 : Product  Inputs=*/  OutDataTypeStr=single  SampleTime=2.08333333333333e-05  SaturateOnIntegerOverflow=on  RndMeth=Zero
  Out1 : Outport
  wires:
  Divide19/1 -> Out1/1
  In2/1 -> Divide19/2
  In1/1 -> Divide19/1

== system AN_Simulink_Model_v1_fil/Auditory Nerve Model/C1 Chirp Filter/Get C1 Coefficients/Divide2 ==
  In1 : Inport
  In2 : Inport  Port=2
  Divide2 : Product  Inputs=*/  OutDataTypeStr=single  SampleTime=2.08333333333333e-05  SaturateOnIntegerOverflow=on  RndMeth=Zero
  Out1 : Outport
  wires:
  Divide2/1 -> Out1/1
  In2/1 -> Divide2/2
  In1/1 -> Divide2/1

== system AN_Simulink_Model_v1_fil/Auditory Nerve Model/C1 Chirp Filter/Get C1 Coefficients/Divide20 ==
  In1 : Inport
  In2 : Inport  Port=2
  Divide20 : Product  Inputs=*/  OutDataTypeStr=single  SampleTime=2.08333333333333e-05  SaturateOnIntegerOverflow=on  RndMeth=Zero
  Out1 : Outport
  wires:
  Divide20/1 -> Out1/1
  In2/1 -> Divide20/2
  In1/1 -> Divide20/1

== system AN_Simulink_Model_v1_fil/Auditory Nerve Model/C1 Chirp Filter/Get C1 Coefficients/Divide21 ==
  In1 : Inport
  In2 : Inport  Port=2
  Divide21 : Product  Inputs=*/  OutDataTypeStr=single  SampleTime=2.08333333333333e-05  SaturateOnIntegerOverflow=on  RndMeth=Zero
  Out1 : Outport
  wires:
  Divide21/1 -> Out1/1
  In2/1 -> Divide21/2
  In1/1 -> Divide21/1

== system AN_Simulink_Model_v1_fil/Auditory Nerve Model/C1 Chirp Filter/Get C1 Coefficients/Divide22 ==
  In1 : Inport
  In2 : Inport  Port=2
  Divide22 : Product  Inputs=*/  OutDataTypeStr=single  SampleTime=2.08333333333333e-05  SaturateOnIntegerOverflow=on  RndMeth=Zero
  Out1 : Outport
  wires:
  Divide22/1 -> Out1/1
  In2/1 -> Divide22/2
  In1/1 -> Divide22/1

== system AN_Simulink_Model_v1_fil/Auditory Nerve Model/C1 Chirp Filter/Get C1 Coefficients/Divide23 ==
  In1 : Inport
  In2 : Inport  Port=2
  Divide23 : Product  Inputs=*/  OutDataTypeStr=single  SampleTime=2.08333333333333e-05  SaturateOnIntegerOverflow=on  RndMeth=Zero
  Out1 : Outport
  wires:
  Divide23/1 -> Out1/1
  In2/1 -> Divide23/2
  In1/1 -> Divide23/1

== system AN_Simulink_Model_v1_fil/Auditory Nerve Model/C1 Chirp Filter/Get C1 Coefficients/Divide3 ==
  In1 : Inport
  In2 : Inport  Port=2
  Divide3 : Product  Inputs=*/  OutDataTypeStr=single  SampleTime=2.08333333333333e-05  SaturateOnIntegerOverflow=on  RndMeth=Zero
  Out1 : Outport
  wires:
  Divide3/1 -> Out1/1
  In2/1 -> Divide3/2
  In1/1 -> Divide3/1

== system AN_Simulink_Model_v1_fil/Auditory Nerve Model/C1 Chirp Filter/Get C1 Coefficients/Divide4 ==
  In1 : Inport
  In2 : Inport  Port=2
  Divide4 : Product  Inputs=*/  OutDataTypeStr=single  SampleTime=2.08333333333333e-05  SaturateOnIntegerOverflow=on  RndMeth=Zero
  Out1 : Outport
  wires:
  Divide4/1 -> Out1/1
  In2/1 -> Divide4/2
  In1/1 -> Divide4/1

== system AN_Simulink_Model_v1_fil/Auditory Nerve Model/C1 Chirp Filter/Get C1 Coefficients/Divide5 ==
  In1 : Inport
  In2 : Inport  Port=2
  Divide5 : Product  Inputs=*/  OutDataTypeStr=single  SampleTime=2.08333333333333e-05  SaturateOnIntegerOverflow=on  RndMeth=Zero
  Out1 : Outport
  wires:
  Divide5/1 -> Out1/1
  In2/1 -> Divide5/2
  In1/1 -> Divide5/1

== system AN_Simulink_Model_v1_fil/Auditory Nerve Model/C1 Chirp Filter/Get C1 Coefficients/Divide6 ==
  In1 : Inport
  In2 : Inport  Port=2
  Divide6 : Product  Inputs=*/  OutDataTypeStr=single  SampleTime=2.08333333333333e-05  SaturateOnIntegerOverflow=on  RndMeth=Zero
  Out1 : Outport
  wires:
  Divide6/1 -> Out1/1
  In2/1 -> Divide6/2
  In1/1 -> Divide6/1

== system AN_Simulink_Model_v1_fil/Auditory Nerve Model/C1 Chirp Filter/Get C1 Coefficients/Divide7 ==
  In1 : Inport
  In2 : Inport  Port=2
  Divide7 : Product  Inputs=*/  OutDataTypeStr=single  SampleTime=2.08333333333333e-05  SaturateOnIntegerOverflow=on  RndMeth=Zero
  Out1 : Outport
  wires:
  Divide7/1 -> Out1/1
  In2/1 -> Divide7/2
  In1/1 -> Divide7/1

== system AN_Simulink_Model_v1_fil/Auditory Nerve Model/C1 Chirp Filter/Get C1 Coefficients/Divide8 ==
  In1 : Inport
  In2 : Inport  Port=2
  Divide8 : Product  Inputs=*/  OutDataTypeStr=single  SampleTime=2.08333333333333e-05  SaturateOnIntegerOverflow=on  RndMeth=Zero
  Out1 : Outport
  wires:
  Divide8/1 -> Out1/1
  In2/1 -> Divide8/2
  In1/1 -> Divide8/1

== system AN_Simulink_Model_v1_fil/Auditory Nerve Model/C1 Chirp Filter/Get C1 Coefficients/Divide9 ==
  In1 : Inport
  In2 : Inport  Port=2
  Divide9 : Product  Inputs=*/  OutDataTypeStr=single  SampleTime=2.08333333333333e-05  SaturateOnIntegerOverflow=on  RndMeth=Zero
  Out1 : Outport
  wires:
  Divide9/1 -> Out1/1
  In2/1 -> Divide9/2
  In1/1 -> Divide9/1

== system AN_Simulink_Model_v1_fil/Auditory Nerve Model/C1 Chirp Filter/Get C1 Coefficients/Gain10_unaryminus ==
  In1 : Inport
  Gain10_unaryminus : UnaryMinus  SampleTime=2.08333333333333e-05
  Out1 : Outport
  wires:
  Gain10_unaryminus/1 -> Out1/1
  In1/1 -> Gain10_unaryminus/1

== system AN_Simulink_Model_v1_fil/Auditory Nerve Model/C1 Chirp Filter/Get C1 Coefficients/Gain11 ==
  In1 : Inport
  Gain11 : Gain  Gain=single(2)
  Out1 : Outport
  wires:
  Gain11/1 -> Out1/1
  In1/1 -> Gain11/1

== system AN_Simulink_Model_v1_fil/Auditory Nerve Model/C1 Chirp Filter/Get C1 Coefficients/Gain12 ==
  In1 : Inport
  Gain12 : Gain  Gain=single(2)
  Out1 : Outport
  wires:
  Gain12/1 -> Out1/1
  In1/1 -> Gain12/1

== system AN_Simulink_Model_v1_fil/Auditory Nerve Model/C1 Chirp Filter/Get C1 Coefficients/Gain13 ==
  In1 : Inport
  Gain13 : Gain  Gain=single(2)
  Out1 : Outport
  wires:
  Gain13/1 -> Out1/1
  In1/1 -> Gain13/1

== system AN_Simulink_Model_v1_fil/Auditory Nerve Model/C1 Chirp Filter/Get C1 Coefficients/Gain14_unaryminus ==
  In1 : Inport
  Gain14_unaryminus : UnaryMinus  SampleTime=2.08333333333333e-05
  Out1 : Outport
  wires:
  Gain14_unaryminus/1 -> Out1/1
  In1/1 -> Gain14_unaryminus/1

== system AN_Simulink_Model_v1_fil/Auditory Nerve Model/C1 Chirp Filter/Get C1 Coefficients/Gain1_unaryminus ==
  In1 : Inport
  Gain1_unaryminus : UnaryMinus  SampleTime=2.08333333333333e-05
  Out1 : Outport
  wires:
  Gain1_unaryminus/1 -> Out1/1
  In1/1 -> Gain1_unaryminus/1

== system AN_Simulink_Model_v1_fil/Auditory Nerve Model/C1 Chirp Filter/Get C1 Coefficients/Gain2_unaryminus ==
  In1 : Inport
  Gain2_unaryminus : UnaryMinus  SampleTime=2.08333333333333e-05
  Out1 : Outport
  wires:
  Gain2_unaryminus/1 -> Out1/1
  In1/1 -> Gain2_unaryminus/1

== system AN_Simulink_Model_v1_fil/Auditory Nerve Model/C1 Chirp Filter/Get C1 Coefficients/Gain3_unaryminus ==
  In1 : Inport
  Gain3_unaryminus : UnaryMinus  SampleTime=2.08333333333333e-05
  Out1 : Outport
  wires:
  Gain3_unaryminus/1 -> Out1/1
  In1/1 -> Gain3_unaryminus/1

== system AN_Simulink_Model_v1_fil/Auditory Nerve Model/C1 Chirp Filter/Get C1 Coefficients/Gain4 ==
  In1 : Inport
  Gain4 : Gain  Gain=single(2)
  Out1 : Outport
  wires:
  Gain4/1 -> Out1/1
  In1/1 -> Gain4/1

== system AN_Simulink_Model_v1_fil/Auditory Nerve Model/C1 Chirp Filter/Get C1 Coefficients/Gain5 ==
  In1 : Inport
  Gain5 : Gain  Gain=single(2)
  Out1 : Outport
  wires:
  Gain5/1 -> Out1/1
  In1/1 -> Gain5/1

== system AN_Simulink_Model_v1_fil/Auditory Nerve Model/C1 Chirp Filter/Get C1 Coefficients/Gain6_unaryminus ==
  In1 : Inport
  Gain6_unaryminus : UnaryMinus  SampleTime=2.08333333333333e-05
  Out1 : Outport
  wires:
  Gain6_unaryminus/1 -> Out1/1
  In1/1 -> Gain6_unaryminus/1

== system AN_Simulink_Model_v1_fil/Auditory Nerve Model/C1 Chirp Filter/Get C1 Coefficients/Gain7 ==
  In1 : Inport
  Gain7 : Gain  Gain=single(-2)
  Out1 : Outport
  wires:
  Gain7/1 -> Out1/1
  In1/1 -> Gain7/1

== system AN_Simulink_Model_v1_fil/Auditory Nerve Model/C1 Chirp Filter/Get C1 Coefficients/Gain9_unaryminus ==
  In1 : Inport
  Gain9_unaryminus : UnaryMinus  SampleTime=2.08333333333333e-05
  Out1 : Outport
  wires:
  Gain9_unaryminus/1 -> Out1/1
  In1/1 -> Gain9_unaryminus/1

== system AN_Simulink_Model_v1_fil/Auditory Nerve Model/C1 Chirp Filter/Get C1 Coefficients/Product28 ==
  In1 : Inport
  In2 : Inport  Port=2
  Product28 : Product  Inputs=**  OutDataTypeStr=single  SampleTime=2.08333333333333e-05
  Out1 : Outport
  wires:
  Product28/1 -> Out1/1
  In2/1 -> Product28/2
  In1/1 -> Product28/1

== system AN_Simulink_Model_v1_fil/Auditory Nerve Model/C1 Chirp Filter/Get C1 Coefficients/Product29 ==
  In1 : Inport
  In2 : Inport  Port=2
  Product29 : Product  Inputs=**  OutDataTypeStr=single  SampleTime=2.08333333333333e-05
  Out1 : Outport
  wires:
  Product29/1 -> Out1/1
  In2/1 -> Product29/2
  In1/1 -> Product29/1

== system AN_Simulink_Model_v1_fil/Auditory Nerve Model/C1 Chirp Filter/Get C1 Coefficients/Product30 ==
  In1 : Inport
  In2 : Inport  Port=2
  Product30 : Product  Inputs=**  OutDataTypeStr=single  SampleTime=2.08333333333333e-05
  Out1 : Outport
  wires:
  Product30/1 -> Out1/1
  In2/1 -> Product30/2
  In1/1 -> Product30/1

== system AN_Simulink_Model_v1_fil/Auditory Nerve Model/C1 Chirp Filter/Get C1 Coefficients/Product34 ==
  In1 : Inport
  In2 : Inport  Port=2
  Product34 : Product  Inputs=**  OutDataTypeStr=single  SampleTime=2.08333333333333e-05
  Out1 : Outport
  wires:
  Product34/1 -> Out1/1
  In2/1 -> Product34/2
  In1/1 -> Product34/1

== system AN_Simulink_Model_v1_fil/Auditory Nerve Model/C1 Chirp Filter/Get C1 Coefficients/Product35 ==
  In1 : Inport
  In2 : Inport  Port=2
  Product35 : Product  Inputs=**  OutDataTypeStr=single  SampleTime=2.08333333333333e-05
  Out1 : Outport
  wires:
  Product35/1 -> Out1/1
  In2/1 -> Product35/2
  In1/1 -> Product35/1

== system AN_Simulink_Model_v1_fil/Auditory Nerve Model/C1 Chirp Filter/Get C1 Coefficients/Product36 ==
  In1 : Inport
  In2 : Inport  Port=2
  Product36 : Product  Inputs=**  OutDataTypeStr=single  SampleTime=2.08333333333333e-05
  Out1 : Outport
  wires:
  Product36/1 -> Out1/1
  In2/1 -> Product36/2
  In1/1 -> Product36/1

== system AN_Simulink_Model_v1_fil/Auditory Nerve Model/C1 Chirp Filter/Get C1 Coefficients/Product37 ==
  In1 : Inport
  In2 : Inport  Port=2
  Product37 : Product  Inputs=**  OutDataTypeStr=single  SampleTime=2.08333333333333e-05
  Out1 : Outport
  wires:
  Product37/1 -> Out1/1
  In2/1 -> Product37/2
  In1/1 -> Product37/1

== system AN_Simulink_Model_v1_fil/Auditory Nerve Model/C1 Chirp Filter/Get C1 Coefficients/Product38 ==
  In1 : Inport
  In2 : Inport  Port=2
  Product38 : Product  Inputs=**  OutDataTypeStr=single  SampleTime=2.08333333333333e-05
  Out1 : Outport
  wires:
  Product38/1 -> Out1/1
  In2/1 -> Product38/2
  In1/1 -> Product38/1

== system AN_Simulink_Model_v1_fil/Auditory Nerve Model/C1 Chirp Filter/Get C1 Coefficients/Product39 ==
  In1 : Inport
  In2 : Inport  Port=2
  Product39 : Product  Inputs=**  OutDataTypeStr=single  SampleTime=2.08333333333333e-05
  Out1 : Outport
  wires:
  Product39/1 -> Out1/1
  In2/1 -> Product39/2
  In1/1 -> Product39/1

== system AN_Simulink_Model_v1_fil/Auditory Nerve Model/C1 Chirp Filter/Get C1 Coefficients/Subtract ==
  In1 : Inport
  In2 : Inport  Port=2
  Subtract : Sum  Inputs=+-  OutDataTypeStr=single  SampleTime=2.08333333333333e-05  SaturateOnIntegerOverflow=on  InputSameDT=on
  Out1 : Outport
  wires:
  Subtract/1 -> Out1/1
  In2/1 -> Subtract/2
  In1/1 -> Subtract/1

== system AN_Simulink_Model_v1_fil/Auditory Nerve Model/C1 Chirp Filter/Get C1 Coefficients/Subtract1 ==
  In1 : Inport
  In2 : Inport  Port=2
  Subtract1 : Sum  Inputs=+-  OutDataTypeStr=single  SampleTime=2.08333333333333e-05  SaturateOnIntegerOverflow=on  InputSameDT=on
  Out1 : Outport
  wires:
  Subtract1/1 -> Out1/1
  In2/1 -> Subtract1/2
  In1/1 -> Subtract1/1

== system AN_Simulink_Model_v1_fil/Auditory Nerve Model/C1 Chirp Filter/Get C1 Coefficients/Subtract10 ==
  In1 : Inport
  In2 : Inport  Port=2
  Subtract10 : Sum  Inputs=+-  OutDataTypeStr=single  SampleTime=2.08333333333333e-05  SaturateOnIntegerOverflow=on  InputSameDT=on
  Out1 : Outport
  wires:
  Subtract10/1 -> Out1/1
  In2/1 -> Subtract10/2
  In1/1 -> Subtract10/1

== system AN_Simulink_Model_v1_fil/Auditory Nerve Model/C1 Chirp Filter/Get C1 Coefficients/Subtract11 ==
  In1 : Inport
  In2 : Inport  Port=2
  Subtract11 : Sum  Inputs=+-  OutDataTypeStr=single  SampleTime=2.08333333333333e-05  SaturateOnIntegerOverflow=on  InputSameDT=on
  Out1 : Outport
  wires:
  Subtract11/1 -> Out1/1
  In2/1 -> Subtract11/2
  In1/1 -> Subtract11/1

== system AN_Simulink_Model_v1_fil/Auditory Nerve Model/C1 Chirp Filter/Get C1 Coefficients/Subtract12 ==
  In1 : Inport
  In2 : Inport  Port=2
  Subtract12 : Sum  Inputs=+-  OutDataTypeStr=single  SampleTime=2.08333333333333e-05  SaturateOnIntegerOverflow=on  InputSameDT=on
  Out1 : Outport
  wires:
  Subtract12/1 -> Out1/1
  In2/1 -> Subtract12/2
  In1/1 -> Subtract12/1

== system AN_Simulink_Model_v1_fil/Auditory Nerve Model/C1 Chirp Filter/Get C1 Coefficients/Subtract13 ==
  In1 : Inport
  In2 : Inport  Port=2
  Subtract13 : Sum  Inputs=+-  OutDataTypeStr=single  SampleTime=2.08333333333333e-05  SaturateOnIntegerOverflow=on  InputSameDT=on
  Out1 : Outport
  wires:
  Subtract13/1 -> Out1/1
  In2/1 -> Subtract13/2
  In1/1 -> Subtract13/1

== system AN_Simulink_Model_v1_fil/Auditory Nerve Model/C1 Chirp Filter/Get C1 Coefficients/Subtract2 ==
  In1 : Inport
  In2 : Inport  Port=2
  Subtract2 : Sum  Inputs=+-  OutDataTypeStr=single  SampleTime=2.08333333333333e-05  SaturateOnIntegerOverflow=on  InputSameDT=on
  Out1 : Outport
  wires:
  Subtract2/1 -> Out1/1
  In2/1 -> Subtract2/2
  In1/1 -> Subtract2/1

== system AN_Simulink_Model_v1_fil/Auditory Nerve Model/C1 Chirp Filter/Get C1 Coefficients/Subtract6 ==
  In1 : Inport
  In2 : Inport  Port=2
  Subtract6 : Sum  Inputs=--  OutDataTypeStr=single  SampleTime=2.08333333333333e-05  SaturateOnIntegerOverflow=on  InputSameDT=on
  Out1 : Outport
  wires:
  Subtract6/1 -> Out1/1
  In2/1 -> Subtract6/2
  In1/1 -> Subtract6/1

== system AN_Simulink_Model_v1_fil/Auditory Nerve Model/C1 Chirp Filter/Get C1 Coefficients/Subtract7 ==
  In1 : Inport
  In2 : Inport  Port=2
  Subtract7 : Sum  Inputs=--  OutDataTypeStr=single  SampleTime=2.08333333333333e-05  SaturateOnIntegerOverflow=on  InputSameDT=on
  Out1 : Outport
  wires:
  Subtract7/1 -> Out1/1
  In2/1 -> Subtract7/2
  In1/1 -> Subtract7/1

== system AN_Simulink_Model_v1_fil/Auditory Nerve Model/C1 Chirp Filter/Get C1 Coefficients/Subtract8 ==
  In1 : Inport
  In2 : Inport  Port=2
  Subtract8 : Sum  Inputs=--  OutDataTypeStr=single  SampleTime=2.08333333333333e-05  SaturateOnIntegerOverflow=on  InputSameDT=on
  Out1 : Outport
  wires:
  Subtract8/1 -> Out1/1
  In2/1 -> Subtract8/2
  In1/1 -> Subtract8/1

== system AN_Simulink_Model_v1_fil/Auditory Nerve Model/C1 Chirp Filter/Get C1 Coefficients/Subtract9 ==
  In1 : Inport
  In2 : Inport  Port=2
  Subtract9 : Sum  Inputs=+-  OutDataTypeStr=single  SampleTime=2.08333333333333e-05  SaturateOnIntegerOverflow=on  InputSameDT=on
  Out1 : Outport
  wires:
  Subtract9/1 -> Out1/1
  In2/1 -> Subtract9/2
  In1/1 -> Subtract9/1

== system AN_Simulink_Model_v1_fil/Auditory Nerve Model/C1 Chirp Filter/Get C1 Coefficients/Trigonometric Function ==
  In1 : Inport
  Trigonometric Function : Trigonometry  Operator=atan  SampleTime=2.08333333333333e-05
  Out1 : Outport
  wires:
  Trigonometric Function/1 -> Out1/1
  In1/1 -> Trigonometric Function/1

== system AN_Simulink_Model_v1_fil/Auditory Nerve Model/C1 Chirp Filter/Get C1 Coefficients/Trigonometric Function1 ==
  In1 : Inport
  Trigonometric Function1 : Trigonometry  Operator=atan  SampleTime=2.08333333333333e-05
  Out1 : Outport
  wires:
  Trigonometric Function1/1 -> Out1/1
  In1/1 -> Trigonometric Function1/1

== system AN_Simulink_Model_v1_fil/Auditory Nerve Model/C1 Chirp Filter/Get C1 Coefficients/Trigonometric Function2 ==
  In1 : Inport
  Trigonometric Function2 : Trigonometry  Operator=atan  SampleTime=2.08333333333333e-05
  Out1 : Outport
  wires:
  Trigonometric Function2/1 -> Out1/1
  In1/1 -> Trigonometric Function2/1

== system AN_Simulink_Model_v1_fil/Auditory Nerve Model/C1 Chirp Filter/Get C1 Coefficients/Trigonometric Function3 ==
  In1 : Inport
  Trigonometric Function3 : Trigonometry  Operator=atan  SampleTime=2.08333333333333e-05
  Out1 : Outport
  wires:
  Trigonometric Function3/1 -> Out1/1
  In1/1 -> Trigonometric Function3/1

== system AN_Simulink_Model_v1_fil/Auditory Nerve Model/C1 Chirp Filter/Get C1 Coefficients/Trigonometric Function4 ==
  In1 : Inport
  Trigonometric Function4 : Trigonometry  Operator=atan  SampleTime=2.08333333333333e-05
  Out1 : Outport
  wires:
  Trigonometric Function4/1 -> Out1/1
  In1/1 -> Trigonometric Function4/1

== system AN_Simulink_Model_v1_fil/Auditory Nerve Model/C1 Chirp Filter/Get C1 Coefficients/Trigonometric Function5 ==
  In1 : Inport
  Trigonometric Function5 : Trigonometry  Operator=atan  SampleTime=2.08333333333333e-05
  Out1 : Outport
  wires:
  Trigonometric Function5/1 -> Out1/1
  In1/1 -> Trigonometric Function5/1

== system AN_Simulink_Model_v1_fil/Auditory Nerve Model/C1 Chirp Filter/Get C1 Coefficients/Trigonometric Function6 ==
  In1 : Inport
  Trigonometric Function6 : Trigonometry  Operator=tan  SampleTime=2.08333333333333e-05
  Out1 : Outport
  wires:
  Trigonometric Function6/1 -> Out1/1
  In1/1 -> Trigonometric Function6/1
